simulink subsystem "rss_ActElecAgElecSpdCmptHybr"  (R2023a)
settings: Solver=VariableStepAuto  StartTime=0.0  StopTime=inf  RelTol=1e-3
undefined symbols (not defined in the file): bit, Cdbl_facPLLCtlKiMaxVal, Cdbl_facPLLCtlKpMaxVal, Cdbl_facVltgIntegFltCoeffMaxVal, Cdbl_indPhIndcMaxVal, Cdbl_indPhIndcPeakVal, Cdbl_iPhCurrMaxVal, Cdbl_iPhCurrPeakVal, Cdbl_nElecAgSpdMaxVal, Cdbl_nElecAgSpdPeakVal, Cdbl_psiPermMagFlxMaxVal, Cdbl_psiPermMagFlxPeakVal, Cdbl_resPhRstnMaxVal, Cdbl_resPhRstnPeakVal, Cdbl_tiMedTaskSmpTi, Cdbl_uPhVltgMaxVal, Cdbl_uSplyVltgPeakVal, dt_Standardize_s16p15b0, dt_Standardize_u16p15b0, ENM_MOTO_STATUS, Gs16_facPLLCtlKp_MAP_nActElecSpd_Y, Gs16_tiSenlElecAgDel_C, Gu16_facFlxObsFltCoeff_C, Gu16_facPLLCtlKi_MAP, Gu16_facPLLCtlKp_MAP, Gu16_indQaxIndc_C, Gu16_resPhRstn_C, Gu8_facPLLCtlKp_MAP_tPCBTempSubs_X, Gu8_numPPNum_C, lb_parOper6MaxVal, lb_parOper7MaxVal
libraries: lib_conversion x25, lib_discrete_time_integrator x5, lib_iir_filter x4, lib_configurable_parameter x3, lib_trigonometric_function x2, lib_finite_difference_derivative x2, simulink x1, lib_discrete_time_PI_controller32bit x1, lib_cart_to_polar_coor_transformer x1, lib_park_transform x1
settings Model: DefaultTestHarness=rss_ActualAngleAndSpeedComputation_thu  Creator=CAV2OFO  LastModifiedBy=xiaoqiang.yuan
settings OptimizationCC: ReuseModelBlockBuffer=off

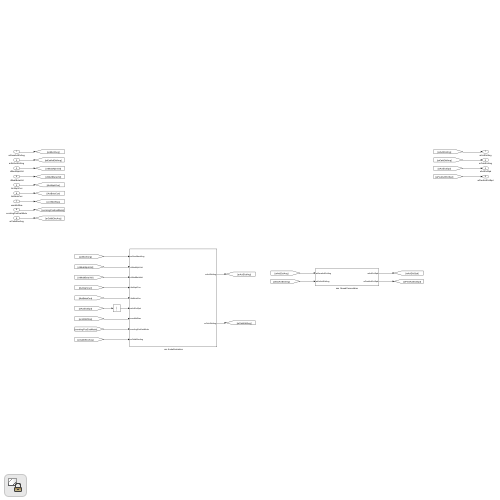
[thumbnail: Simulink's stored preview of the top-level diagram]
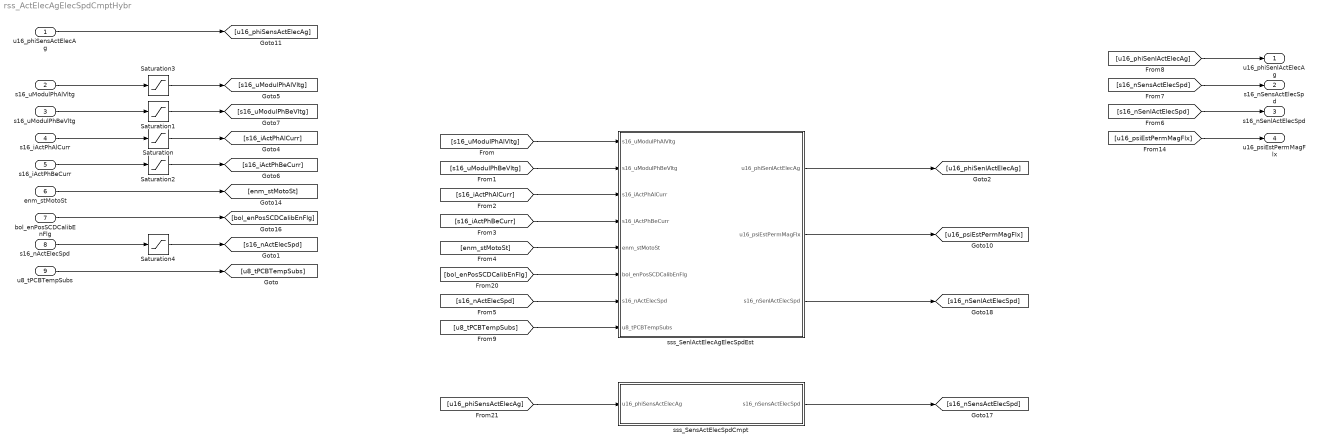
== system rss_ActElecAgElecSpdCmptHybr ==
  u16_phiSensActElecAg : Inport  OutDataTypeStr=dt_RadAng_u16r15b0
  s16_uModulPhAlVltg : Inport  Port=2  OutDataTypeStr=dt_Standardize_s16p15b0
  s16_uModulPhBeVltg : Inport  Port=3  OutDataTypeStr=dt_Standardize_s16p15b0
  s16_iActPhAlCurr : Inport  Port=4  OutDataTypeStr=dt_Standardize_s16p15b0
  s16_iActPhBeCurr : Inport  Port=5  OutDataTypeStr=dt_Standardize_s16p15b0
  enm_stMotoSt : Inport  Port=6  OutDataTypeStr=Enum: ENM_MOTO_STATUS
  bol_enPosSCDCalibEnFlg : Inport  Port=7  OutDataTypeStr=boolean
  s16_nActElecSpd : Inport  Port=8
  u8_tPCBTempSubs : Inport  Port=9
  Saturation : Saturate  UpperLimit=Cdbl_iPhCurrMaxVal  LowerLimit=-Cdbl_iPhCurrMaxVal
  Saturation1 : Saturate  UpperLimit=Cdbl_uPhVltgMaxVal  LowerLimit=-Cdbl_uPhVltgMaxVal
  Saturation2 : Saturate  UpperLimit=Cdbl_iPhCurrMaxVal  LowerLimit=-Cdbl_iPhCurrMaxVal
  Saturation3 : Saturate  UpperLimit=Cdbl_uPhVltgMaxVal  LowerLimit=-Cdbl_uPhVltgMaxVal
  Saturation4 : Saturate  UpperLimit=Cdbl_nElecAgSpdMaxVal  LowerLimit=-Cdbl_nElecAgSpdMaxVal
  sss_SenlActElecAgElecSpdEst : Subsystem
  sss_SensActElecSpdCmpt : Subsystem
  u16_phiSenlActElecAg : Outport  OutDataTypeStr=dt_RadAng_u16r15b0
  s16_nSensActElecSpd : Outport  Port=2  OutDataTypeStr=dt_Standardize_s16p15b0
  s16_nSenlActElecSpd : Outport  Port=3  OutDataTypeStr=dt_Standardize_s16p15b0  PortDimensions=1  VectorParamsAs1DForOutWhenUnconnected=off
  u16_psiEstPermMagFlx : Outport  Port=4  OutDataTypeStr=dt_Standardize_u16p15b0  PortDimensions=1  VectorParamsAs1DForOutWhenUnconnected=off
  wires:
  [s16_uModulPhAlVltg] -> sss_SenlActElecAgElecSpdEst/1(s16_uModulPhAlVltg)
  [s16_iActPhBeCurr] -> sss_SenlActElecAgElecSpdEst/4(s16_iActPhBeCurr)
  s16_iActPhBeCurr/1 -> Saturation2/1
  s16_iActPhAlCurr/1 -> Saturation/1
  [s16_iActPhAlCurr] -> sss_SenlActElecAgElecSpdEst/3(s16_iActPhAlCurr)
  sss_SenlActElecAgElecSpdEst/2(u16_psiEstPermMagFlx) -> [u16_psiEstPermMagFlx]
  [u16_psiEstPermMagFlx] -> u16_psiEstPermMagFlx/1
  [s16_uModulPhBeVltg] -> sss_SenlActElecAgElecSpdEst/2(s16_uModulPhBeVltg)
  s16_uModulPhBeVltg/1 -> Saturation1/1
  [u16_phiSenlActElecAg] -> u16_phiSenlActElecAg/1
  s16_uModulPhAlVltg/1 -> Saturation3/1
  [s16_nSensActElecSpd] -> s16_nSensActElecSpd/1
  enm_stMotoSt/1 -> [enm_stMotoSt]
  [enm_stMotoSt] -> sss_SenlActElecAgElecSpdEst/5(enm_stMotoSt)
  sss_SenlActElecAgElecSpdEst/1(u16_phiSenlActElecAg) -> [u16_phiSenlActElecAg]
  [s16_nSenlActElecSpd] -> s16_nSenlActElecSpd/1
  u16_phiSensActElecAg/1 -> [u16_phiSensActElecAg]
  bol_enPosSCDCalibEnFlg/1 -> [bol_enPosSCDCalibEnFlg]
  [bol_enPosSCDCalibEnFlg] -> sss_SenlActElecAgElecSpdEst/6(bol_enPosSCDCalibEnFlg)
  Saturation3/1 -> [s16_uModulPhAlVltg]
  Saturation1/1 -> [s16_uModulPhBeVltg]
  Saturation/1 -> [s16_iActPhAlCurr]
  Saturation2/1 -> [s16_iActPhBeCurr]
  [u16_phiSensActElecAg] -> sss_SensActElecSpdCmpt/1(u16_phiSensActElecAg)
  sss_SensActElecSpdCmpt/1(s16_nSensActElecSpd) -> [s16_nSensActElecSpd]
  sss_SenlActElecAgElecSpdEst/3(s16_nSenlActElecSpd) -> [s16_nSenlActElecSpd]
  s16_nActElecSpd/1 -> Saturation4/1
  [s16_nActElecSpd] -> sss_SenlActElecAgElecSpdEst/7(s16_nActElecSpd)
  Saturation4/1 -> [s16_nActElecSpd]
  [u8_tPCBTempSubs] -> sss_SenlActElecAgElecSpdEst/8(u8_tPCBTempSubs)
  u8_tPCBTempSubs/1 -> [u8_tPCBTempSubs]

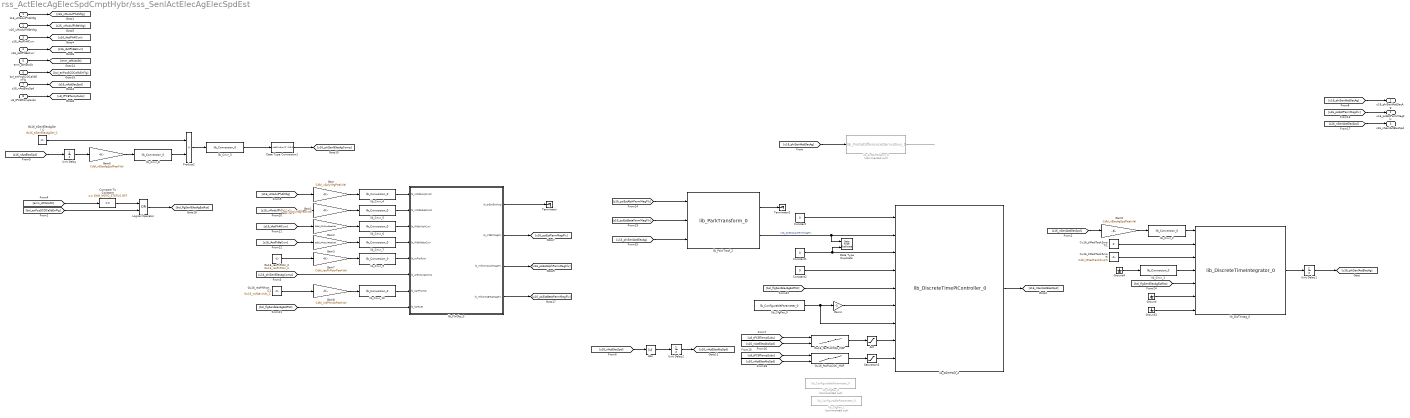
== system rss_ActElecAgElecSpdCmptHybr/sss_SenlActElecAgElecSpdEst ==
  s16_uModulPhAlVltg : Inport
  s16_uModulPhBeVltg : Inport  Port=2
  s16_iActPhAlCurr : Inport  Port=3
  s16_iActPhBeCurr : Inport  Port=4
  enm_stMotoSt : Inport  Port=5
  bol_enPosSCDCalibEnFlg : Inport  Port=6
  s16_nActElecSpd : Inport  Port=7
  u8_tPCBTempSubs : Inport  Port=8
  Abs : Abs  SaturateOnIntegerOverflow=off
  Ast : Saturate  UpperLimit=Cdbl_facPLLCtlKpMaxVal  LowerLimit=0
  Compare To Constant : simulink/Logic and Bit Operations/Compare To Constant  relop===  const=ENM_MOTO_STATUS.OFF  OutDataTypeStr=boolean
  Constant : Constant  Value=0  OutDataTypeStr=dt_Standardize_s16p15b0
  Constant1 : Constant  Value=0  OutDataTypeStr=Inherit: Inherit via back propagation
  Constant2 : Constant  Value=0  OutDataTypeStr=dt_Standardize_s16p15b0
  Cu16_tiMedTaskSmpTi : Constant  Value=Cdbl_tiMedTaskSmpTi
  Cu16_tiMedTaskSmpTi1 : Constant  Value=0  OutDataTypeStr=dt_RadAng_u16r15b0
  Data Type Duplicate : DataTypeDuplicate
  Data Type Conversion1 : DataTypeConversion  OutDataTypeStr=fixdt(0,16,pi*2^-15,0)  SaturateOnIntegerOverflow=off  RndMeth=Floor
  Gain : Gain  Gain=Cdbl_uSplyVltgPeakVal  OutDataTypeStr=Inherit: Inherit via back propagation
  Gain1 : Gain  Gain=Cdbl_uSplyVltgPeakVal  OutDataTypeStr=Inherit: Inherit via back propagation
  Gain2 : Gain  Gain=Cdbl_iPhCurrPeakVal  OutDataTypeStr=Inherit: Inherit via back propagation
  Gain3 : Gain  Gain=Cdbl_iPhCurrPeakVal  OutDataTypeStr=Inherit: Inherit via back propagation
  Gain4 : Gain  Gain=-1  OutDataTypeStr=Inherit: Same as input
  Gain5 : Gain  Gain=Cdbl_nElecAgSpdPeakVal  OutDataTypeStr=Inherit: Inherit via back propagation
  Gain6 : Gain  Gain=Cdbl_nElecAgSpdPeakVal  OutDataTypeStr=Inherit: Inherit via back propagation
  Gain7 : Gain  Gain=Cdbl_resPhRstnPeakVal  OutDataTypeStr=Inherit: Inherit via back propagation
  Gain8 : Gain  Gain=Cdbl_indPhIndcPeakVal  OutDataTypeStr=Inherit: Inherit via back propagation
  Ground : Ground
  Ground1 : Ground
  Ground4 : Ground
  Gs16_tiSenlElecAgDel_C : Constant  Value=Gs16_tiSenlElecAgDel_C
  Gu16_facPLLCtlKi_MAP : Lookup_n-D  BreakpointsForDimension1=Gu8_facPLLCtlKp_MAP_tPCBTempSubs_X  BreakpointsForDimension2=Gs16_facPLLCtlKp_MAP_nActElecSpd_Y  Table=Gu16_facPLLCtlKi_MAP  ExtrapMethod=Clip  InternalRulePriority=Speed  OutDataTypeStr=Inherit: Inherit from 'Table data'  RndMeth=Simplest  InputSameDT=off
      settings: InputPortMap=u0,u1
  Gu16_facPLLCtlKp_MAP : Lookup_n-D  BreakpointsForDimension1=Gu8_facPLLCtlKp_MAP_tPCBTempSubs_X  BreakpointsForDimension2=Gs16_facPLLCtlKp_MAP_nActElecSpd_Y  Table=Gu16_facPLLCtlKp_MAP  ExtrapMethod=Clip  InternalRulePriority=Speed  OutDataTypeStr=Inherit: Inherit from 'Table data'  RndMeth=Simplest  InputSameDT=off
      settings: InputPortMap=u0,u1
  Gu16_resPhRstn_C : Constant  Value=Gu16_resPhRstn_C
  Gu16_resPhRstn_C1 : Constant  Value=Gu16_indQaxIndc_C
  Logical Operator : Logic  Operator=OR  AllPortsSameDT=off  OutDataTypeStr=boolean
  Product2 : Product  OutDataTypeStr=Inherit: Inherit via back propagation
  Saturation3 : Saturate  UpperLimit=Cdbl_facPLLCtlKiMaxVal  LowerLimit=0
  Terminator : Terminator
  Terminator2 : Terminator
  Unit Delay : UnitDelay  SampleTime=-1  HasFrameUpgradeWarning=on
  Unit Delay1 : UnitDelay  SampleTime=-1  HasFrameUpgradeWarning=on
  Unit Delay2 : UnitDelay  SampleTime=-1  HasFrameUpgradeWarning=on
  lib_CfgPar_0 : lib_configurable_parameter/lib_ConfigurableParameter_0  lb_parCnfgPar=Gs16_nPLLElecAgSpdUpLim_C  lb_parDataType=Inherit: Inherit from 'Constant value'  lb_parUpLim=Cdbl_nElecAgSpdMaxVal  lb_parLowLim=0
  lib_CfgPar_1 : lib_configurable_parameter/lib_ConfigurableParameter_0  Commented=on  lb_parCnfgPar=Gu16_facPLLCtlKp_C  lb_parDataType=Inherit: Inherit from 'Constant value'  lb_parUpLim=Cdbl_facPLLCtlKpMaxVal  lb_parLowLim=0
  lib_CfgPar_2 : lib_configurable_parameter/lib_ConfigurableParameter_0  Commented=on  lb_parCnfgPar=Gu16_facPLLCtlKi_C  lb_parDataType=Inherit: Inherit from 'Constant value'  lb_parUpLim=Cdbl_facPLLCtlKiMaxVal  lb_parLowLim=0
  lib_Cnvr_1 : lib_conversion/lib_Conversion_0  lb_parDataType=uint8  lb_parOutpMaxVal=[]  lb_parOutpMinVal=[]  lb_parSatFlag=off
  lib_Cnvr_10 : lib_conversion/lib_Conversion_0  lb_parDataType=fixdt(0,16)  lb_parOutpMaxVal=Cdbl_indPhIndcPeakVal  lb_parOutpMinVal=[]  RndMeth=Simplest  lb_parSatFlag=off
  lib_Cnvr_2 : lib_conversion/lib_Conversion_0  lb_parDataType=fixdt(1,16)  lb_parOutpMaxVal=Cdbl_nElecAgSpdPeakVal  lb_parOutpMinVal=[]  RndMeth=Simplest  lb_parSatFlag=off
  lib_Cnvr_3 : lib_conversion/lib_Conversion_0  lb_parDataType=fixdt(1,16,pi*2^-15,0)  lb_parOutpMaxVal=[]  lb_parOutpMinVal=[]  lb_parSatFlag=off
  lib_Cnvr_4 : lib_conversion/lib_Conversion_0  lb_parDataType=fixdt(1,16)  lb_parOutpMaxVal=Cdbl_uSplyVltgPeakVal  lb_parOutpMinVal=[]  RndMeth=Simplest  lb_parSatFlag=off
  lib_Cnvr_5 : lib_conversion/lib_Conversion_0  lb_parDataType=fixdt(1,16)  lb_parOutpMaxVal=Cdbl_uSplyVltgPeakVal  lb_parOutpMinVal=[]  RndMeth=Simplest  lb_parSatFlag=off
  lib_Cnvr_6 : lib_conversion/lib_Conversion_0  lb_parDataType=fixdt(1,16)  lb_parOutpMaxVal=Cdbl_iPhCurrPeakVal  lb_parOutpMinVal=[]  RndMeth=Simplest  lb_parSatFlag=off
  lib_Cnvr_7 : lib_conversion/lib_Conversion_0  lb_parDataType=fixdt(1,16)  lb_parOutpMaxVal=Cdbl_iPhCurrPeakVal  lb_parOutpMinVal=[]  RndMeth=Simplest  lb_parSatFlag=off
  lib_Cnvr_8 : lib_conversion/lib_Conversion_0  lb_parDataType=fixdt(1,16)  lb_parOutpMaxVal=Cdbl_nElecAgSpdPeakVal  lb_parOutpMinVal=[]  RndMeth=Simplest  lb_parSatFlag=off
  lib_Cnvr_9 : lib_conversion/lib_Conversion_0  lb_parDataType=fixdt(0,16)  lb_parOutpMaxVal=Cdbl_resPhRstnPeakVal  lb_parOutpMinVal=[]  RndMeth=Simplest  lb_parSatFlag=off
  lib_DisTiInteg_0 : lib_discrete_time_integrator/lib_DiscreteTimeIntegrator_0  lb_parMaxInpVal=Cdbl_nElecAgSpdMaxVal*Cdbl_nElecAgSpdPeakVal  lb_parMinInpVal=-Cdbl_nElecAgSpdMaxVal*Cdbl_nElecAgSpdPeakVal  lb_parMaxSampTime=double(Cdbl_tiMedTaskSmpTi)  lb_parMaxIntgGain=0  lb_parAccmDataTypeMode=Same of output  lb_parOutpDataType=dt_RadAng_u16r15b0  lb_parIntgScopMode=Angular signal  lb_parSatFlag=off
  lib_DisTiPICtl_2 : lib_discrete_time_PI_controller32bit/lib_DiscreteTimePIController_0  lb_parSampTime=Cdbl_tiMedTaskSmpTi  lb_parMaxSampTime=0.1  lb_parMaxPropGain=Cdbl_facPLLCtlKpMaxVal  lb_parMaxIntgGain=Cdbl_facPLLCtlKiMaxVal  lb_parRefInpMaxVal=Cdbl_psiPermMagFlxMaxVal  lb_parRefInpMinVal=-Cdbl_psiPermMagFlxMaxVal  lb_parMaxErrVal=2*Cdbl_psiPermMagFlxMaxVal  lb_parMinErrVal=-2*Cdbl_psiPermMagFlxMaxVal  lb_parMaxOutpVal=Cdbl_nElecAgSpdMaxVal  lb_parMinOutpVal=-Cdbl_nElecAgSpdMaxVal  lb_parAccmDataTypeMode=32-bit  lb_parOutpDataType=dt_Standardize_s16p15b0  lb_parSatMode=anti-windup with back-calculation
  lib_FlxObs_0 : Subsystem  mask{lb_parPhsRstnMaxVal=Cdbl_resPhRstnMaxVal*Cdbl_resPhRstnPeakVal, lb_parPhsIndcMaxVal=Cdbl_indPhIndcMaxVal*Cdbl_indPhIndcPeakVal, lb_parPhsCurrMaxVal=Cdbl_iPhCurrMaxVal*Cdbl_iPhCurrPeakVal, lb_parPhsVoltMaxVal=Cdbl_uPhVltgMaxVal*Cdbl_uSplyVltgPeakVal, lb_parVoltIntgMaxVal=Cdbl_psiPermMagFlxMaxVal*Cdbl_psiPermMagFlxPeakVal*10, lb_parEstMagFluxMaxVal=Cdbl_psiPermMagFlxMaxVal*Cdbl_psiPermMagFlxPeakVal, lb_parPolePairNum=Gu8_numPPNum_C, lb_parSampTime=Cdbl_tiMedTaskSmpTi, lb_parFiltCoef=Gu16_facFlxObsFltCoeff_C, lb_parFltrCoefMaxVal=Cdbl_facVltgIntegFltCoeffMaxVal, lb_fluxPeak=Cdbl_psiPermMagFlxPeakVal, lb_parFluxAmpDataType=dt_Standardize_u16p15b0, lb_parFluxDataType=dt_Standardize_s16p15b0, lb_parBitNumMode=16-bit}
      mask prompts: lb_parPhsRstnMaxVal "Maximum phase resistance [Ohm]:"; lb_parPhsIndcMaxVal "Maximum phase inductance [H]:"; lb_parPhsCurrMaxVal "Maximum phase current [A]:"; lb_parPhsVoltMaxVal "Maximum phase voltage [V]:"; lb_parVoltIntgMaxVal "Maximum value for voltage integrator [Wb]:"; lb_parEstMagFluxMaxVal "Maximum estimated magnet flux [Wb]:"; lb_parPolePairNum "Number of pole pairs:"; lb_parSampTime "Sampling time [s]:"; lb_parFiltCoef "High-pass filter coefficient:"; lb_parFltrCoefMaxVal "High-pass filter coefficient maximum value:"; lb_fluxPeak "Peak output physical value[Wb]:"; lb_parFluxAmpDataType "Permanent magnet flux amplitude data type:"; lb_parFluxDataType "Permanent magnet flux data type:"; lb_parBitNumMode "Bits number for internal calculations:"
      mask init:
      | switch lb_parBitNumMode
      |     case '16-bit'
      |         lb_parBitNum = 16;
      |     case '32-bit'
      |         lb_parBitNum = 32;
      |     otherwise
      |         lb_parBitNum = 16;
      | end
      | 
      | % Operation 1: R*I
      | lb_parOper1MaxVal = lb_parPhsRstnMaxVal*lb_parPhsCurrMaxVal;
      | 
      | % Operation 2: V-R*I
      | lb_parOper2MaxVal = lb_parPhsVoltMaxVal+lb_parPhsRstnMaxVal*lb_parPhsCurrMaxVal;
      | 
      | % Operation 3: L*I
      | lb_parOper3MaxVal = lb_parPhsIndcMaxVal*lb_parPhsCurrMaxVal;
      | 
      | % Operation 4: integral of V-R*I
      | temp.oper4MaxVal = lb_parOper3MaxVal+lb_parEstMagFluxMaxVal;
      | lb_parIntgTurnOnThrs = lb_parVoltIntgMaxVal/2;
      | temp.intgMaxVal = lb_parVoltIntgMaxVal;
      | temp.NumType = fi(temp.intgMaxVal,1,lb_parBitNum);
      | lb_parIntgSlopExp = temp.NumType.FractionLength;
      | 
      | % Operation 5: filtering of flux
      | temp.NumType = fi(lb_parEstMagFluxMaxVal,1,16);
      | lb_parFiltSlopExp = temp.NumType.FractionLength;
      | 
      | % Operation 6: psi*I
      | %lb_parOper6MaxVal = lb_parPhsCurrMaxVal*lb_parEstMagFluxMaxVal;
      | 
      | % Operation 7: 2*psi*I
      | %lb_parOper7MaxVal = 2*lb_parPhsCurrMaxVal*lb_parEstMagFluxMaxVal;
      | 
      | % Operation 8: 3/2*Np
      | %lb_parOper8MaxVal = 3/2*double(lb_parPolePairNum);
      settings: LibrarySourceBlock=lib_flux_observer/lib_FluxObserver_0
      mask TypeOptions lb_parBitNumMode: 16-bit | 32-bit
      mask DialogControl DescGroupVar Prompt: Current Coupling block
      mask DialogControl DescTextVar Prompt: This block estimates electric angle, Permenant magnet flux and electric torque
      mask DialogControl modlPar Prompt: Model Parameters
      mask DialogControl Container3_copy Prompt: Data type:
      mask DialogControl Container3 Prompt: Operating modes:
  lib_FntDiffFltDrvt_0 : lib_finite_difference_derivative/lib_FiniteDifferenceDerivative_0  Commented=on  lb_parSampTime=Cdbl_tiMedTaskSmpTi  lb_parMaxInpVar=Cdbl_phiMaxMedTaskElecAgVrnt  lb_parOutpPhyPek=Cdbl_nElecAgSpdPeakVal  lb_parAngInpMode=on  lb_parOutpDataType=dt_Standardize_s16p15b0
      link override vss_AngleModeSelection: VariantControlMode=label  LabelModeActiveChoice=lb_parAngInpModeLbl
  lib_ParkTrasf_2 : lib_park_transform/lib_ParkTransform_0  VariantControl=ClarkTransf_MIL_flo  lb_parSelRotFrmeAxis=d-axis
  u16_phiSenlActElecAg : Outport
  u16_psiEstPermMagFlx : Outport  Port=2
  s16_nSenlActElecSpd : Outport  Port=3
  wires:
  Saturation3/1 -> lib_DisTiPICtl_2/9
  Ast/1 -> lib_DisTiPICtl_2/8
  [s16_nActElecAbsSpd] -> Gu16_facPLLCtlKi_MAP/2
  [s16_nActElecAbsSpd] -> Gu16_facPLLCtlKp_MAP/2
  Unit Delay2/1 -> [s16_nActElecAbsSpd]
  Gu16_facPLLCtlKi_MAP/1 -> Saturation3/1
  Gu16_facPLLCtlKp_MAP/1 -> Ast/1
  [u8_tPCBTempSubs] -> Gu16_facPLLCtlKi_MAP/1
  u8_tPCBTempSubs/1 -> [u8_tPCBTempSubs]
  [u8_tPCBTempSubs] -> Gu16_facPLLCtlKp_MAP/1
  Abs/1 -> Unit Delay2/1
  [s16_nActElecSpd] -> Abs/1
  [u16_phiSenlActElecAg] -> lib_FntDiffFltDrvt_0/1
  lib_FntDiffFltDrvt_0/1 -> ?
  s16_nActElecSpd/1 -> [s16_nActElecSpd]
  lib_FlxObs_0/4(lb_mfCompBetaMagFlx) -> [s16_psiEstBetaPermMagFlx]
  lib_FlxObs_0/3(lb_mfCompAlphMagFlx) -> [s16_psiEstAlphPermMagFlx]
  lib_Cnvr_10/1 -> lib_FlxObs_0/7(lb_parPhsIndc)
  Gain8/1 -> lib_Cnvr_10/1
  Gu16_resPhRstn_C1/1 -> Gain8/1
  Gu16_resPhRstn_C/1 -> Gain7/1
  lib_Cnvr_9/1 -> lib_FlxObs_0/5(lb_rsPhsRstn)
  Gain7/1 -> lib_Cnvr_9/1
  Unit Delay/1 -> Gain6/1
  lib_Cnvr_8/1 -> Product2/2
  Gain6/1 -> lib_Cnvr_8/1
  lib_DisTiPICtl_2/1 -> [s16_nSenlActElecSpd]
  Unit Delay1/1 -> [u16_phiSenlActElecAg]
  lib_Cnvr_2/1 -> lib_DisTiInteg_0/1
  Gain5/1 -> lib_Cnvr_2/1
  [s16_nSenlActElecSpd] -> Gain5/1
  Gain4/1 -> lib_DisTiPICtl_2/6
  lib_CfgPar_0/1 -> Gain4/1, lib_DisTiPICtl_2/7
  Ground1/1 -> lib_DisTiInteg_0/7
  Ground/1 -> lib_DisTiInteg_0/6
  [bol_flgSenlElecAgEstRst] -> lib_DisTiInteg_0/5
  lib_Cnvr_1/1 -> lib_DisTiInteg_0/4
  Cu16_tiMedTaskSmpTi1/1 -> lib_DisTiInteg_0/2
  Cu16_tiMedTaskSmpTi/1 -> lib_DisTiInteg_0/3
  Ground4/1 -> lib_Cnvr_1/1
  lib_DisTiInteg_0/1 -> Unit Delay1/1
  [bol_flgSenlElecAgEstRst] -> lib_DisTiPICtl_2/5
  [bol_flgSenlElecAgEstRst] -> lib_FlxObs_0/8(lb_bolRset)
  Logical Operator/1 -> [bol_flgSenlElecAgEstRst]
  Constant2/1 -> lib_DisTiPICtl_2/4
  Constant1/1 -> lib_DisTiPICtl_2/3, Data Type Duplicate/2
  lib_ParkTrasf_2/2 -> lib_DisTiPICtl_2/2, Data Type Duplicate/1  "s16_psiEstQaxPermMagFlx"
  lib_ParkTrasf_2/1 -> Terminator2/1
  Constant/1 -> lib_DisTiPICtl_2/1
  [u16_phiSenlActElecAg] -> lib_ParkTrasf_2/3
  [s16_psiEstBetaPermMagFlx] -> lib_ParkTrasf_2/2
  [s16_psiEstAlphPermMagFlx] -> lib_ParkTrasf_2/1
  [s16_nActElecSpd] -> Unit Delay/1
  [s16_nSenlActElecSpd] -> s16_nSenlActElecSpd/1
  [bol_enPosSCDCalibEnFlg] -> Logical Operator/2
  Compare To Constant/1 -> Logical Operator/1
  [u16_phiSenlElecAgComp] -> lib_FlxObs_0/6(lb_arElctAngComp)
  [s16_iActPhBeCurr] -> Gain3/1
  lib_Cnvr_4/1 -> lib_FlxObs_0/1(lb_vtFdbkAlphVolt)
  [s16_uModulPhAlVltg] -> Gain/1
  Gain3/1 -> lib_Cnvr_7/1
  lib_FlxObs_0/1(lb_arEstElctAng) -> Terminator/1
  lib_FlxObs_0/2(lb_mfEstMagFlx) -> [u16_psiEstPermMagFlx]
  [s16_iActPhAlCurr] -> Gain2/1
  Gain1/1 -> lib_Cnvr_5/1
  lib_Cnvr_6/1 -> lib_FlxObs_0/3(lb_iFdbkAlphCurr)
  Gain2/1 -> lib_Cnvr_6/1
  Gain/1 -> lib_Cnvr_4/1
  lib_Cnvr_7/1 -> lib_FlxObs_0/4(lb_iFdbkBetaCurr)
  [enm_stMotoSt] -> Compare To Constant/1
  lib_Cnvr_5/1 -> lib_FlxObs_0/2(lb_vtFdbkBetaVolt)
  [s16_uModulPhBeVltg] -> Gain1/1
  bol_enPosSCDCalibEnFlg/1 -> [bol_enPosSCDCalibEnFlg]
  s16_uModulPhBeVltg/1 -> [s16_uModulPhBeVltg]
  s16_uModulPhAlVltg/1 -> [s16_uModulPhAlVltg]
  enm_stMotoSt/1 -> [enm_stMotoSt]
  lib_Cnvr_3/1 -> Data Type Conversion1/1
  Data Type Conversion1/1 -> [u16_phiSenlElecAgComp]
  Product2/1 -> lib_Cnvr_3/1
  Gs16_tiSenlElecAgDel_C/1 -> Product2/1
  [u16_psiEstPermMagFlx] -> u16_psiEstPermMagFlx/1
  [u16_phiSenlActElecAg] -> u16_phiSenlActElecAg/1
  s16_iActPhBeCurr/1 -> [s16_iActPhBeCurr]
  s16_iActPhAlCurr/1 -> [s16_iActPhAlCurr]

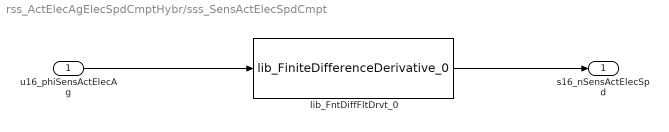
== system rss_ActElecAgElecSpdCmptHybr/sss_SensActElecSpdCmpt ==
  u16_phiSensActElecAg : Inport
  lib_FntDiffFltDrvt_0 : lib_finite_difference_derivative/lib_FiniteDifferenceDerivative_0  lb_parSampTime=Cdbl_tiMedTaskSmpTi  lb_parMaxInpVar=Cdbl_phiMaxMedTaskElecAgVrnt  lb_parOutpPhyPek=Cdbl_nElecAgSpdPeakVal  lb_parAngInpMode=on  lb_parOutpDataType=dt_Standardize_s16p15b0
      link override vss_AngleModeSelection: VariantControlMode=label  LabelModeActiveChoice=lb_parAngInpModeLbl
  s16_nSensActElecSpd : Outport
  wires:
  lib_FntDiffFltDrvt_0/1 -> s16_nSensActElecSpd/1
  u16_phiSensActElecAg/1 -> lib_FntDiffFltDrvt_0/1

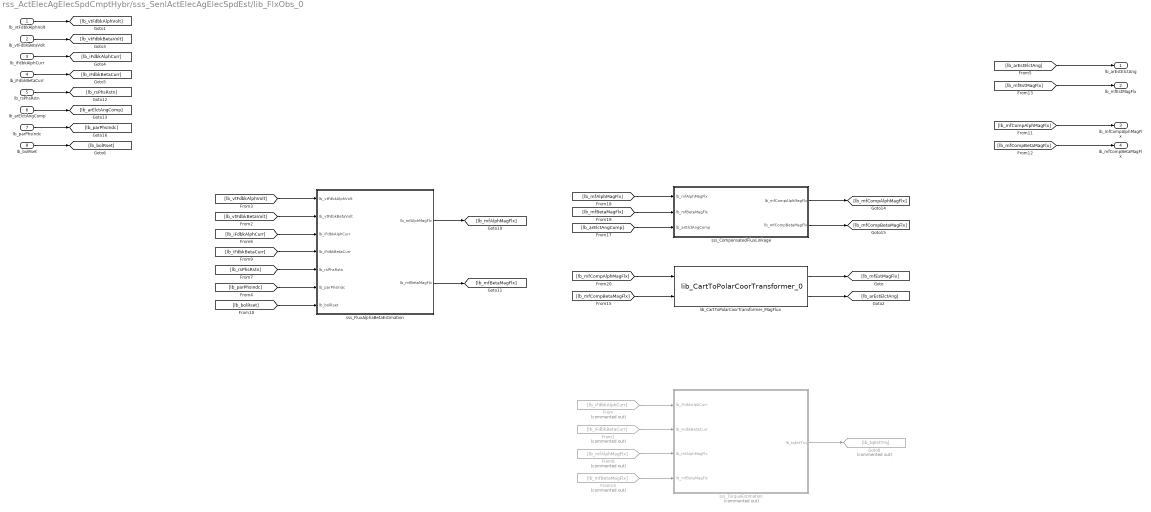
== system rss_ActElecAgElecSpdCmptHybr/sss_SenlActElecAgElecSpdEst/lib_FlxObs_0 ==
  lb_vtFdbkAlphVolt : Inport
  lb_vtFdbkBetaVolt : Inport  Port=2
  lb_iFdbkAlphCurr : Inport  Port=3
  lb_iFdbkBetaCurr : Inport  Port=4
  lb_rsPhsRstn : Inport  Port=5
  lb_arElctAngComp : Inport  Port=6  OutDataTypeStr=fixdt(0,16,pi*2^-15,0)
  lb_parPhsIndc : Inport  Port=7
  lb_bolRset : Inport  Port=8
  From : From  Commented=on  GotoTag=lb_iFdbkAlphCurr
  From1 : From  Commented=on  GotoTag=lb_iFdbkBetaCurr
  From14 : From  Commented=on  GotoTag=lb_mfBetaMagFlx
  From8 : From  Commented=on  GotoTag=lb_mfAlphMagFlx
  Goto8 : Goto  Commented=on  GotoTag=lb_tqEstTrq
  lib_CartToPolarCoorTransformer_MagFlux : lib_cart_to_polar_coor_transformer/lib_CartToPolarCoorTransformer_0  lb_parAsinLktSize=4095  lb_parAmpLktSize=512  lb_parOutpAmpDataType=lb_parFluxAmpDataType
      link override lib_MagnitudeCalculator_1/Compare To Constant/Compare: Operator===  OutDataTypeStr=boolean
      link override lib_MagnitudeCalculator_1/Compare To Constant1/Compare: Operator===  OutDataTypeStr=boolean
  sss_CompensatedFluxLinkage : Subsystem
  sss_FluxAlphaBetaEstimation : Subsystem
  sss_TorqueEstimation : Subsystem  Commented=on
  lb_arEstElctAng : Outport
  lb_mfEstMagFlx : Outport  Port=2
  lb_mfCompAlphMagFlx : Outport  Port=3
  lb_mfCompBetaMagFlx : Outport  Port=4
  wires:
  sss_CompensatedFluxLinkage/2(lb_mfCompBetaMagFlx) -> [lb_mfCompBetaMagFlx]
  sss_CompensatedFluxLinkage/1(lb_mfCompAlphMagFlx) -> [lb_mfCompAlphMagFlx]
  [lb_parPhsIndc] -> sss_FluxAlphaBetaEstimation/6(lb_parPhsIndc)
  lb_parPhsIndc/1 -> [lb_parPhsIndc]
  [lb_mfCompBetaMagFlx] -> lb_mfCompBetaMagFlx/1
  [lb_mfCompAlphMagFlx] -> lb_mfCompAlphMagFlx/1
  [lb_bolRset] -> sss_FluxAlphaBetaEstimation/7(lb_bolRset)
  lb_bolRset/1 -> [lb_bolRset]
  [lb_mfBetaMagFlx] -> sss_CompensatedFluxLinkage/2(lb_mfBetaMagFlx)
  [lb_mfAlphMagFlx] -> sss_CompensatedFluxLinkage/1(lb_mfAlphMagFlx)
  [lb_arElctAngComp] -> sss_CompensatedFluxLinkage/3(lb_arElctAngComp)
  lb_arElctAngComp/1 -> [lb_arElctAngComp]
  [lb_rsPhsRstn] -> sss_FluxAlphaBetaEstimation/5(lb_rsPhsRstn)
  lb_rsPhsRstn/1 -> [lb_rsPhsRstn]
  [lb_mfCompAlphMagFlx] -> lib_CartToPolarCoorTransformer_MagFlux/1
  [lb_mfCompBetaMagFlx] -> lib_CartToPolarCoorTransformer_MagFlux/2
  lib_CartToPolarCoorTransformer_MagFlux/2 -> [lb_arEstElctAng]
  From1/1 -> sss_TorqueEstimation/2(lb_iFdbkBetaCurr)
  From/1 -> sss_TorqueEstimation/1(lb_iFdbkAlphCurr)
  From14/1 -> sss_TorqueEstimation/4(lb_mfBetaMagFlx)
  From8/1 -> sss_TorqueEstimation/3(lb_mfAlphMagFlx)
  sss_FluxAlphaBetaEstimation/2(lb_mfBetaMagFlx) -> [lb_mfBetaMagFlx]
  sss_FluxAlphaBetaEstimation/1(lb_mfAlphMagFlx) -> [lb_mfAlphMagFlx]
  [lb_iFdbkBetaCurr] -> sss_FluxAlphaBetaEstimation/4(lb_iFdbkBetaCurr)
  [lb_vtFdbkBetaVolt] -> sss_FluxAlphaBetaEstimation/2(lb_vtFdbkBetaVolt)
  [lb_vtFdbkAlphVolt] -> sss_FluxAlphaBetaEstimation/1(lb_vtFdbkAlphVolt)
  lib_CartToPolarCoorTransformer_MagFlux/1 -> [lb_mfEstMagFlx]
  [lb_arEstElctAng] -> lb_arEstElctAng/1
  [lb_iFdbkAlphCurr] -> sss_FluxAlphaBetaEstimation/3(lb_iFdbkAlphCurr)
  lb_iFdbkAlphCurr/1 -> [lb_iFdbkAlphCurr]
  lb_vtFdbkBetaVolt/1 -> [lb_vtFdbkBetaVolt]
  sss_TorqueEstimation/1(lb_tqEstTrq) -> Goto8/1
  [lb_mfEstMagFlx] -> lb_mfEstMagFlx/1
  lb_iFdbkBetaCurr/1 -> [lb_iFdbkBetaCurr]
  lb_vtFdbkAlphVolt/1 -> [lb_vtFdbkAlphVolt]

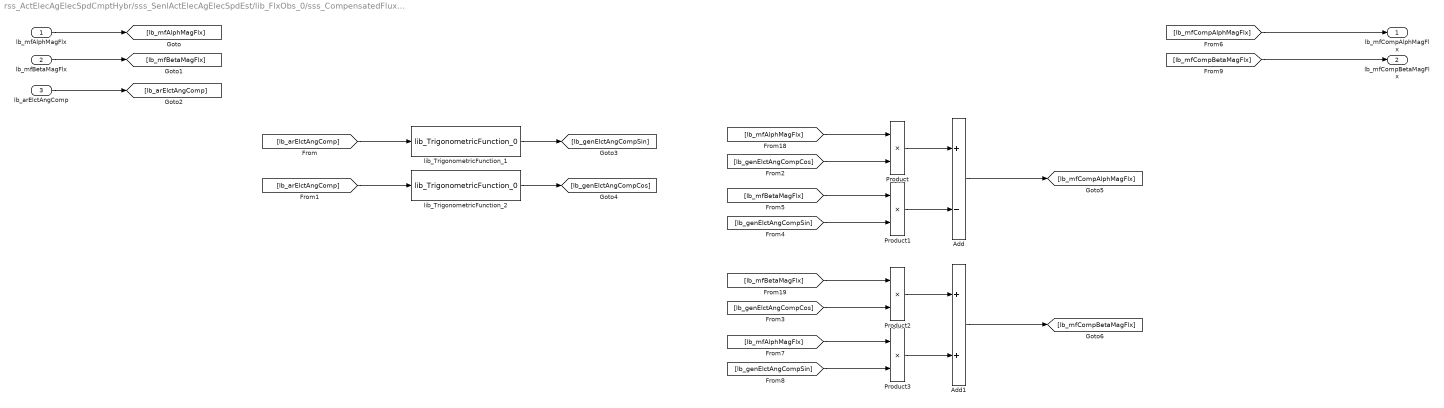
== system rss_ActElecAgElecSpdCmptHybr/sss_SenlActElecAgElecSpdEst/lib_FlxObs_0/sss_CompensatedFluxLinkage ==
  lb_mfAlphMagFlx : Inport
  lb_mfBetaMagFlx : Inport  Port=2
  lb_arElctAngComp : Inport  Port=3
  Add : Sum  Inputs=+-  OutDataTypeStr=Inherit: Same as first input
  Add1 : Sum  OutDataTypeStr=Inherit: Same as first input
  Product{,1..3} (4 alike) : Product  OutDataTypeStr=Inherit: Same as first input
  lib_TrigonometricFunction_1 : lib_trigonometric_function/lib_TrigonometricFunction_0  lb_parSelSigType=Sine  lb_parLktSizeStr=1024  lb_parOutpDataType=fixdt(1,16,2^-14,0)
  lib_TrigonometricFunction_2 : lib_trigonometric_function/lib_TrigonometricFunction_0  lb_parSelSigType=Cosine  lb_parLktSizeStr=1024  lb_parOutpDataType=fixdt(1,16,2^-14,0)
  lb_mfCompAlphMagFlx : Outport
  lb_mfCompBetaMagFlx : Outport  Port=2
  wires:
  [lb_mfCompBetaMagFlx] -> lb_mfCompBetaMagFlx/1
  [lb_mfCompAlphMagFlx] -> lb_mfCompAlphMagFlx/1
  Product2/1 -> Add1/1
  [lb_mfBetaMagFlx] -> Product2/1
  Product3/1 -> Add1/2
  Add1/1 -> [lb_mfCompBetaMagFlx]
  [lb_genElctAngCompSin] -> Product3/2
  [lb_genElctAngCompCos] -> Product2/2
  [lb_mfAlphMagFlx] -> Product3/1
  Add/1 -> [lb_mfCompAlphMagFlx]
  Product/1 -> Add/1
  Product1/1 -> Add/2
  [lb_mfBetaMagFlx] -> Product1/1
  [lb_genElctAngCompSin] -> Product1/2
  [lb_genElctAngCompCos] -> Product/2
  [lb_mfAlphMagFlx] -> Product/1
  lib_TrigonometricFunction_2/1 -> [lb_genElctAngCompCos]
  lib_TrigonometricFunction_1/1 -> [lb_genElctAngCompSin]
  [lb_arElctAngComp] -> lib_TrigonometricFunction_2/1
  [lb_arElctAngComp] -> lib_TrigonometricFunction_1/1
  lb_arElctAngComp/1 -> [lb_arElctAngComp]
  lb_mfBetaMagFlx/1 -> [lb_mfBetaMagFlx]
  lb_mfAlphMagFlx/1 -> [lb_mfAlphMagFlx]

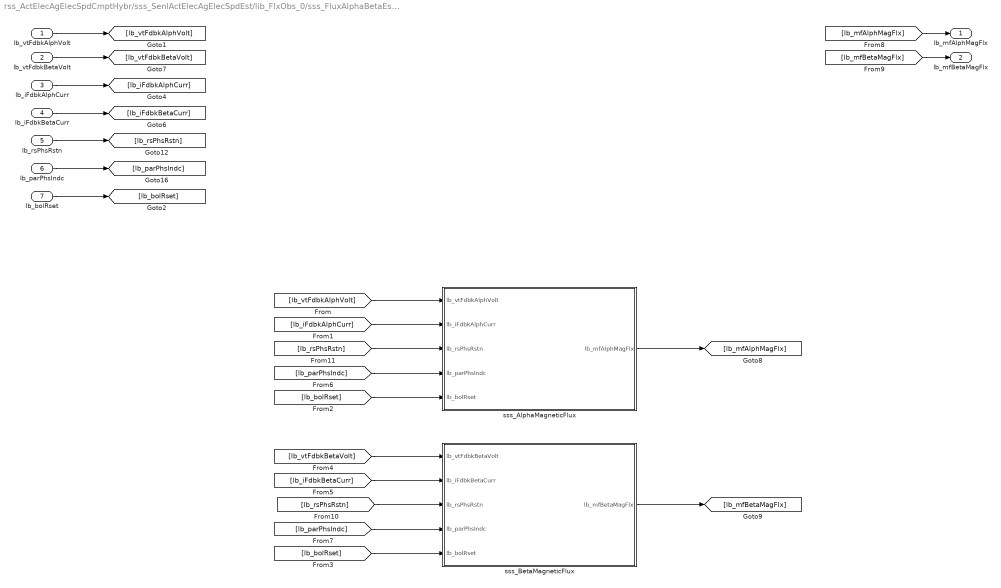
== system rss_ActElecAgElecSpdCmptHybr/sss_SenlActElecAgElecSpdEst/lib_FlxObs_0/sss_FluxAlphaBetaEstimation ==
  lb_vtFdbkAlphVolt : Inport
  lb_vtFdbkBetaVolt : Inport  Port=2
  lb_iFdbkAlphCurr : Inport  Port=3
  lb_iFdbkBetaCurr : Inport  Port=4
  lb_rsPhsRstn : Inport  Port=5
  lb_parPhsIndc : Inport  Port=6
  lb_bolRset : Inport  Port=7
  sss_AlphaMagneticFlux : Subsystem
  sss_BetaMagneticFlux : Subsystem
  lb_mfAlphMagFlx : Outport
  lb_mfBetaMagFlx : Outport  Port=2
  wires:
  [lb_parPhsIndc] -> sss_BetaMagneticFlux/4(lb_parPhsIndc)
  [lb_parPhsIndc] -> sss_AlphaMagneticFlux/4(lb_parPhsIndc)
  lb_parPhsIndc/1 -> [lb_parPhsIndc]
  [lb_bolRset] -> sss_BetaMagneticFlux/5(lb_bolRset)
  [lb_bolRset] -> sss_AlphaMagneticFlux/5(lb_bolRset)
  lb_bolRset/1 -> [lb_bolRset]
  sss_BetaMagneticFlux/1(lb_mfBetaMagFlx) -> [lb_mfBetaMagFlx]
  [lb_rsPhsRstn] -> sss_AlphaMagneticFlux/3(lb_rsPhsRstn)
  [lb_rsPhsRstn] -> sss_BetaMagneticFlux/3(lb_rsPhsRstn)
  lb_rsPhsRstn/1 -> [lb_rsPhsRstn]
  [lb_mfBetaMagFlx] -> lb_mfBetaMagFlx/1
  [lb_mfAlphMagFlx] -> lb_mfAlphMagFlx/1
  lb_vtFdbkBetaVolt/1 -> [lb_vtFdbkBetaVolt]
  lb_iFdbkBetaCurr/1 -> [lb_iFdbkBetaCurr]
  [lb_vtFdbkBetaVolt] -> sss_BetaMagneticFlux/1(lb_vtFdbkBetaVolt)
  [lb_iFdbkBetaCurr] -> sss_BetaMagneticFlux/2(lb_iFdbkBetaCurr)
  sss_AlphaMagneticFlux/1(lb_mfAlphMagFlx) -> [lb_mfAlphMagFlx]
  [lb_iFdbkAlphCurr] -> sss_AlphaMagneticFlux/2(lb_iFdbkAlphCurr)
  [lb_vtFdbkAlphVolt] -> sss_AlphaMagneticFlux/1(lb_vtFdbkAlphVolt)
  lb_vtFdbkAlphVolt/1 -> [lb_vtFdbkAlphVolt]
  lb_iFdbkAlphCurr/1 -> [lb_iFdbkAlphCurr]

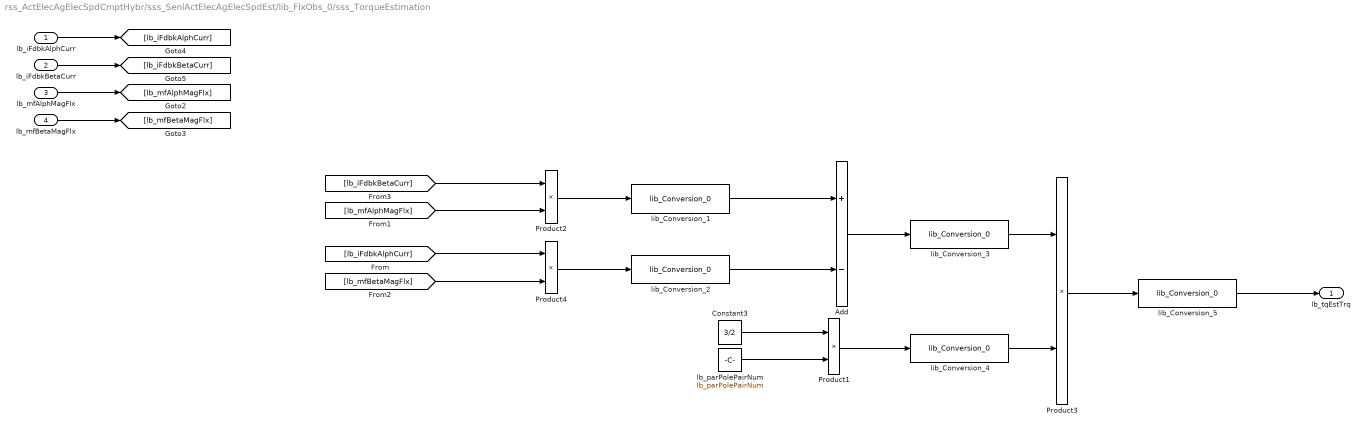
== system rss_ActElecAgElecSpdCmptHybr/sss_SenlActElecAgElecSpdEst/lib_FlxObs_0/sss_TorqueEstimation ==
  lb_iFdbkAlphCurr : Inport
  lb_iFdbkBetaCurr : Inport  Port=2
  lb_mfAlphMagFlx : Inport  Port=3
  lb_mfBetaMagFlx : Inport  Port=4
  Add : Sum  Inputs=+-  OutDataTypeStr=Inherit: Inherit via back propagation
  Constant3 : Constant  Value=3/2  OutDataTypeStr=fixdt(0,16,2^-15,0)
  Product{1..4} (4 alike) : Product  OutDataTypeStr=Inherit: Inherit via back propagation
  lb_parPolePairNum : Constant  Value=lb_parPolePairNum
  lib_Conversion_1 : lib_conversion/lib_Conversion_0  lb_parDataType=fixdt(1,16)  lb_parOutpMaxVal=lb_parOper6MaxVal  lb_parOutpMinVal=-lb_parOper6MaxVal  lb_parSatFlag=off
  lib_Conversion_2 : lib_conversion/lib_Conversion_0  lb_parDataType=fixdt(1,16)  lb_parOutpMaxVal=lb_parOper6MaxVal  lb_parOutpMinVal=-lb_parOper6MaxVal  lb_parSatFlag=off
  lib_Conversion_3 : lib_conversion/lib_Conversion_0  lb_parDataType=fixdt(1,16)  lb_parOutpMaxVal=lb_parOper7MaxVal  lb_parOutpMinVal=-lb_parOper7MaxVal  lb_parSatFlag=off
  lib_Conversion_4 : lib_conversion/lib_Conversion_0  lb_parDataType=fixdt(0,16)  lb_parOutpMaxVal=lb_parOper8MaxVal  lb_parOutpMinVal=[]  lb_parSatFlag=off
  lib_Conversion_5 : lib_conversion/lib_Conversion_0  lb_parDataType=lb_parMotTrqDataType  lb_parOutpMaxVal=[]  lb_parOutpMinVal=[]  lb_parSatFlag=off
  lb_tqEstTrq : Outport
  wires:
  lib_Conversion_2/1 -> Add/2
  Product4/1 -> lib_Conversion_2/1
  lib_Conversion_3/1 -> Product3/1
  lib_Conversion_4/1 -> Product3/2
  Product2/1 -> lib_Conversion_1/1
  lib_Conversion_1/1 -> Add/1
  Product1/1 -> lib_Conversion_4/1
  [lb_iFdbkBetaCurr] -> Product2/1
  [lb_mfAlphMagFlx] -> Product2/2
  [lb_iFdbkAlphCurr] -> Product4/1
  lb_iFdbkBetaCurr/1 -> [lb_iFdbkBetaCurr]
  lb_iFdbkAlphCurr/1 -> [lb_iFdbkAlphCurr]
  lb_parPolePairNum/1 -> Product1/2
  Constant3/1 -> Product1/1
  Add/1 -> lib_Conversion_3/1
  [lb_mfBetaMagFlx] -> Product4/2
  lib_Conversion_5/1 -> lb_tqEstTrq/1
  lb_mfBetaMagFlx/1 -> [lb_mfBetaMagFlx]
  lb_mfAlphMagFlx/1 -> [lb_mfAlphMagFlx]
  Product3/1 -> lib_Conversion_5/1

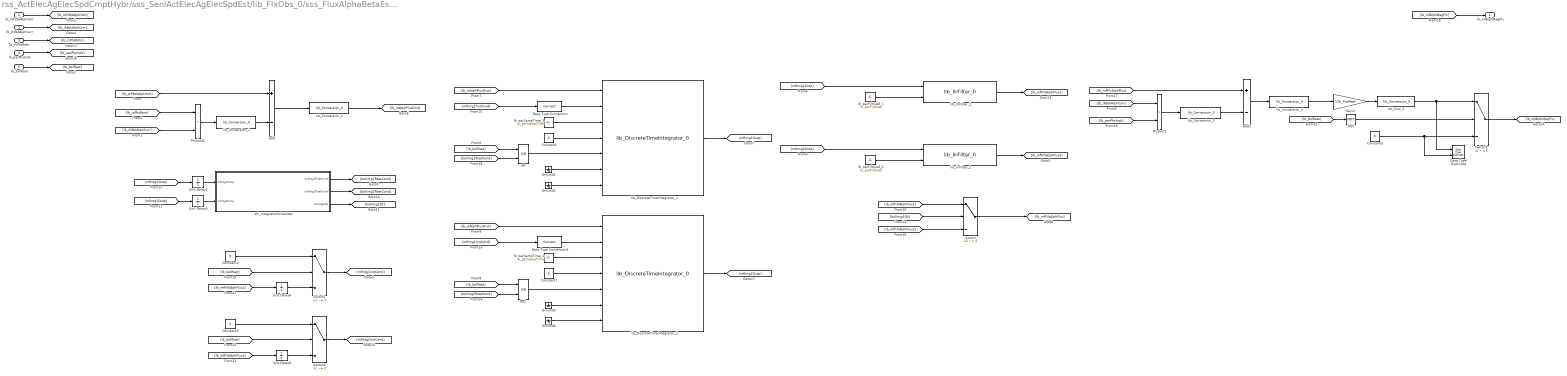
== system rss_ActElecAgElecSpdCmptHybr/sss_SenlActElecAgElecSpdEst/lib_FlxObs_0/sss_FluxAlphaBetaEstimation/sss_AlphaMagneticFlux ==
  lb_vtFdbkAlphVolt : Inport
  lb_iFdbkAlphCurr : Inport  Port=2
  lb_rsPhsRstn : Inport  Port=3
  lb_parPhsIndc : Inport  Port=4
  lb_bolRset : Inport  Port=5
  Add : Sum  Inputs=+-  OutDataTypeStr=Inherit: Inherit via back propagation
  Add1 : Sum  Inputs=+-  OutDataTypeStr=Inherit: Inherit via back propagation
  Constant : Constant  Value=0  OutDataTypeStr=uint8
  Constant1 : Constant  Value=0  OutDataTypeStr=uint8
  Constant2 : Constant  Value=0  OutDataTypeStr=fixdt(1,16,2^-lb_parFiltSlopExp,0)
  Constant3 : Constant  Value=0  OutDataTypeStr=fixdt(1,16,2^-lb_parFiltSlopExp,0)
  Constant5 : Constant  Value=0  OutDataTypeStr=Inherit: Inherit via back propagation
  Data Type Duplicate : DataTypeDuplicate
  Data Type Conversion : DataTypeConversion  SaturateOnIntegerOverflow=off  RndMeth=Floor
  Data Type Conversion1 : DataTypeConversion  SaturateOnIntegerOverflow=off  RndMeth=Floor
  Gain2 : Gain  Gain=1/lb_fluxPeak  OutDataTypeStr=Inherit: Inherit via back propagation
  Ground{1..4} (4 alike) : Ground
  NOT : Logic  Operator=NOT  AllPortsSameDT=off  OutDataTypeStr=boolean
  OR : Logic  Operator=OR  AllPortsSameDT=off  OutDataTypeStr=boolean
  OR1 : Logic  Operator=OR  AllPortsSameDT=off  OutDataTypeStr=boolean
  Product1 : Product  OutDataTypeStr=Inherit: Inherit via back propagation
  Product2 : Product  OutDataTypeStr=Inherit: Inherit via back propagation
  Switch{,1..3} (4 alike) : Switch  Criteria=u2 ~= 0  SaturateOnIntegerOverflow=off  InputSameDT=off
  Unit Delay{2..5} (4 alike) : UnitDelay  SampleTime=-1  HasFrameUpgradeWarning=on
  lb_parFiltCoef_1 : Constant  Value=lb_parFiltCoef
  lb_parFiltCoef_2 : Constant  Value=lb_parFiltCoef
  lb_parSampTime_1 : Constant  Value=lb_parSampTime
  lb_parSampTime_2 : Constant  Value=lb_parSampTime
  lib_Cnvr_1 : lib_conversion/lib_Conversion_0  lb_parDataType=lb_parFluxDataType  lb_parOutpMaxVal=[]  lb_parOutpMinVal=[]  lb_parSatFlag=off
  lib_Conversion_1 : lib_conversion/lib_Conversion_0  lb_parDataType=fixdt(1,lb_parBitNum)  lb_parOutpMaxVal=lb_parOper1MaxVal  lb_parOutpMinVal=-lb_parOper1MaxVal  lb_parSatFlag=off
  lib_Conversion_2 : lib_conversion/lib_Conversion_0  lb_parDataType=fixdt(1,lb_parBitNum)  lb_parOutpMaxVal=lb_parOper2MaxVal  lb_parOutpMinVal=-lb_parOper2MaxVal  lb_parSatFlag=off
  lib_Conversion_3 : lib_conversion/lib_Conversion_0  lb_parDataType=fixdt(1,lb_parBitNum)  lb_parOutpMaxVal=lb_parOper3MaxVal  lb_parOutpMinVal=-lb_parOper3MaxVal  lb_parSatFlag=off
  lib_Conversion_4 : lib_conversion/lib_Conversion_0  lb_parDataType=fixdt(1,16)  lb_parOutpMaxVal=lb_parEstMagFluxMaxVal  lb_parOutpMinVal=-lb_parEstMagFluxMaxVal  lb_parSatFlag=off
  lib_DiscreteTimeIntegrator_1 : lib_discrete_time_integrator/lib_DiscreteTimeIntegrator_0  lb_parMaxInpVal=lb_parOper2MaxVal  lb_parMinInpVal=-lb_parOper2MaxVal  lb_parMaxSampTime=double(lb_parSampTime)  lb_parMaxIntgGain=0  lb_parAccmDataTypeMode=Same of output  lb_parOutpDataType=fixdt(1,lb_parBitNum,2^-lb_parIntgSlopExp,0)  lb_parIntgScopMode=Generic signal  lb_parSatFlag=off
  lib_DiscreteTimeIntegrator_2 : lib_discrete_time_integrator/lib_DiscreteTimeIntegrator_0  lb_parMaxInpVal=lb_parOper2MaxVal  lb_parMinInpVal=-lb_parOper2MaxVal  lb_parMaxSampTime=double(lb_parSampTime)  lb_parMaxIntgGain=0  lb_parAccmDataTypeMode=Same of output  lb_parOutpDataType=fixdt(1,lb_parBitNum,2^-lb_parIntgSlopExp,0)  lb_parIntgScopMode=Generic signal  lb_parSatFlag=off
  lib_IirFilter_1 : lib_iir_filter/lib_IirFilter_0  lb_parMaxInpVal=lb_parVoltIntgMaxVal  lb_parFltrCoefMaxVal=lb_parFltrCoefMaxVal  lb_parBitNumMode=16-bit  lb_parOutpDataType=fixdt(1,16,2^-lb_parFiltSlopExp,0)  lb_parFiltTypeMode=High-pass
      link override vss_FilterVariant: VariantControlMode=label  LabelModeActiveChoice=lb_parHighPassModeLbl
  lib_IirFilter_2 : lib_iir_filter/lib_IirFilter_0  lb_parMaxInpVal=lb_parVoltIntgMaxVal  lb_parFltrCoefMaxVal=lb_parFltrCoefMaxVal  lb_parBitNumMode=16-bit  lb_parOutpDataType=fixdt(1,16,2^-lb_parFiltSlopExp,0)  lb_parFiltTypeMode=High-pass
      link override vss_FilterVariant: VariantControlMode=label  LabelModeActiveChoice=lb_parHighPassModeLbl
  sfc_IntegratorScheduler : Stateflow chart  TreatAsAtomicUnit=on
  lb_mfAlphMagFlx : Outport
  wires:
  [bolIntg2RsetCond] -> OR1/2
  [lb_bolRset] -> OR1/1
  OR1/1 -> lib_DiscreteTimeIntegrator_2/5
  [bolIntg1RsetCond] -> OR/2
  [lb_bolRset] -> OR/1
  OR/1 -> lib_DiscreteTimeIntegrator_1/5
  [lb_vtAlphFluxDrvt] -> lib_DiscreteTimeIntegrator_2/1
  [mfIntg2InitCond] -> Data Type Conversion1/1
  lb_parSampTime_2/1 -> lib_DiscreteTimeIntegrator_2/3
  Data Type Conversion1/1 -> lib_DiscreteTimeIntegrator_2/2
  lib_DiscreteTimeIntegrator_2/1 -> [mfIntg2Outp]
  Ground3/1 -> lib_DiscreteTimeIntegrator_2/6
  Ground4/1 -> lib_DiscreteTimeIntegrator_2/7
  Constant1/1 -> lib_DiscreteTimeIntegrator_2/4
  Switch/1 -> [lb_mfFiltAlphFlux]
  [bolIntg1Ok] -> Switch/2
  [lb_mfFiltAlphFlux1] -> Switch/1
  [lb_mfFiltAlphFlux2] -> Switch/3
  lb_parFiltCoef_2/1 -> lib_IirFilter_2/2
  lib_IirFilter_2/1 -> [lb_mfFiltAlphFlux2]
  [mfIntg2Outp] -> lib_IirFilter_2/1
  [lb_mfFiltAlphFlux1] -> Unit Delay5/1
  Switch1/1 -> [mfIntg1InitCond]
  Constant3/1 -> Switch2/1
  [lb_bolRset] -> Switch2/2
  [lb_bolRset] -> Switch1/2
  Unit Delay5/1 -> Switch2/3
  [lb_mfFiltAlphFlux2] -> Unit Delay4/1
  Constant2/1 -> Switch1/1
  Unit Delay4/1 -> Switch1/3
  Switch2/1 -> [mfIntg2InitCond]
  [mfIntg1Outp] -> Unit Delay2/1
  sfc_IntegratorScheduler/2(bolIntg2RsetCond) -> [bolIntg2RsetCond]
  sfc_IntegratorScheduler/1(bolIntg1RsetCond) -> [bolIntg1RsetCond]
  [mfIntg2Outp] -> Unit Delay3/1
  Unit Delay3/1 -> sfc_IntegratorScheduler/2(mfIntg2Outp)
  sfc_IntegratorScheduler/3(bolIntg1Ok) -> [bolIntg1Ok]
  Unit Delay2/1 -> sfc_IntegratorScheduler/1(mfIntg1Outp)
  Switch3/1 -> [lb_mfAlphMagFlx]
  [lb_vtAlphFluxDrvt] -> lib_DiscreteTimeIntegrator_1/1
  lb_parPhsIndc/1 -> [lb_parPhsIndc]
  lib_Conversion_4/1 -> Gain2/1
  lib_Cnvr_1/1 -> Switch3/1, Data Type Duplicate/1
  Gain2/1 -> lib_Cnvr_1/1
  NOT/1 -> Switch3/2
  Constant5/1 -> Switch3/3, Data Type Duplicate/2
  [lb_bolRset] -> NOT/1
  lb_bolRset/1 -> [lb_bolRset]
  [lb_mfAlphMagFlx] -> lb_mfAlphMagFlx/1
  [mfIntg1InitCond] -> Data Type Conversion/1
  [lb_mfFiltAlphFlux] -> Add1/1
  [mfIntg1Outp] -> lib_IirFilter_1/1
  lib_DiscreteTimeIntegrator_1/1 -> [mfIntg1Outp]
  lib_Conversion_2/1 -> [lb_vtAlphFluxDrvt]
  lib_IirFilter_1/1 -> [lb_mfFiltAlphFlux1]
  lb_parFiltCoef_1/1 -> lib_IirFilter_1/2
  Data Type Conversion/1 -> lib_DiscreteTimeIntegrator_1/2
  lib_Conversion_3/1 -> Add1/2
  Ground2/1 -> lib_DiscreteTimeIntegrator_1/7
  Constant/1 -> lib_DiscreteTimeIntegrator_1/4
  Ground1/1 -> lib_DiscreteTimeIntegrator_1/6
  lb_parSampTime_1/1 -> lib_DiscreteTimeIntegrator_1/3
  lib_Conversion_1/1 -> Add/2
  lb_rsPhsRstn/1 -> [lb_rsPhsRstn]
  Product1/1 -> lib_Conversion_1/1
  Add/1 -> lib_Conversion_2/1
  [lb_vtFdbkAlphVolt] -> Add/1
  lb_vtFdbkAlphVolt/1 -> [lb_vtFdbkAlphVolt]
  lb_iFdbkAlphCurr/1 -> [lb_iFdbkAlphCurr]
  [lb_iFdbkAlphCurr] -> Product1/2
  [lb_parPhsIndc] -> Product2/2
  [lb_rsPhsRstn] -> Product1/1
  [lb_iFdbkAlphCurr] -> Product2/1
  Product2/1 -> lib_Conversion_3/1
  Add1/1 -> lib_Conversion_4/1

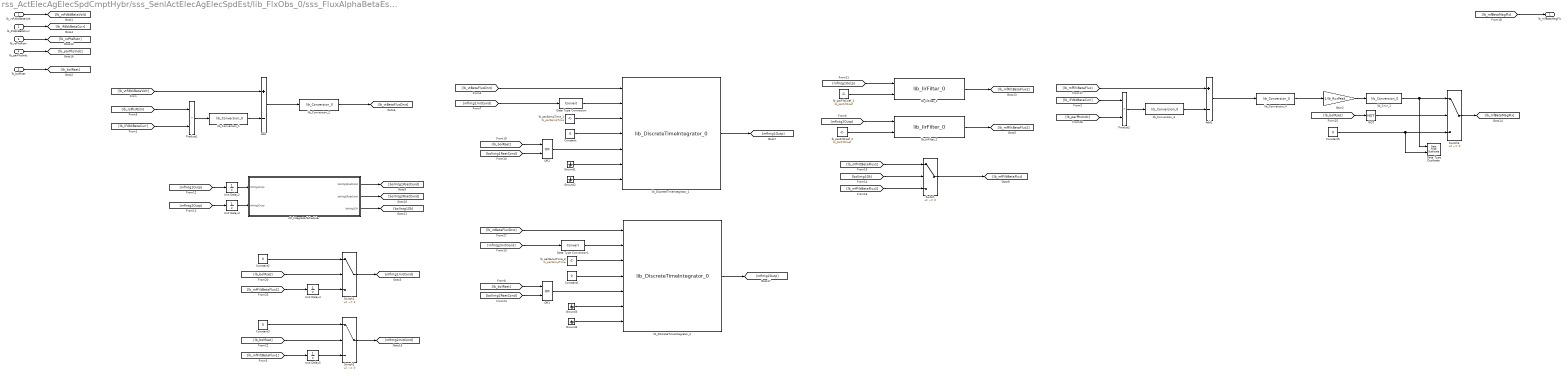
== system rss_ActElecAgElecSpdCmptHybr/sss_SenlActElecAgElecSpdEst/lib_FlxObs_0/sss_FluxAlphaBetaEstimation/sss_BetaMagneticFlux ==
  lb_vtFdbkBetaVolt : Inport
  lb_iFdbkBetaCurr : Inport  Port=2
  lb_rsPhsRstn : Inport  Port=3
  lb_parPhsIndc : Inport  Port=4
  lb_bolRset : Inport  Port=5
  Add : Sum  Inputs=+-  OutDataTypeStr=Inherit: Inherit via back propagation
  Add1 : Sum  Inputs=+-  OutDataTypeStr=Inherit: Inherit via back propagation
  Constant : Constant  Value=0  OutDataTypeStr=uint8
  Constant1 : Constant  Value=0  OutDataTypeStr=uint8
  Constant2 : Constant  Value=0  OutDataTypeStr=fixdt(1,16,2^-lb_parFiltSlopExp,0)
  Constant3 : Constant  Value=0  OutDataTypeStr=fixdt(1,16,2^-lb_parFiltSlopExp,0)
  Constant5 : Constant  Value=0  OutDataTypeStr=Inherit: Inherit via back propagation
  Data Type Duplicate : DataTypeDuplicate
  Data Type Conversion : DataTypeConversion  SaturateOnIntegerOverflow=off  RndMeth=Floor
  Data Type Conversion1 : DataTypeConversion  SaturateOnIntegerOverflow=off  RndMeth=Floor
  Gain2 : Gain  Gain=1/lb_fluxPeak  OutDataTypeStr=Inherit: Inherit via back propagation
  Ground{1..4} (4 alike) : Ground
  NOT : Logic  Operator=NOT  AllPortsSameDT=off  OutDataTypeStr=boolean
  OR1 : Logic  Operator=OR  AllPortsSameDT=off  OutDataTypeStr=boolean
  OR2 : Logic  Operator=OR  AllPortsSameDT=off  OutDataTypeStr=boolean
  Product1 : Product  OutDataTypeStr=Inherit: Inherit via back propagation
  Product2 : Product  OutDataTypeStr=Inherit: Inherit via back propagation
  Switch{,1..3} (4 alike) : Switch  Criteria=u2 ~= 0  SaturateOnIntegerOverflow=off  InputSameDT=off
  Unit Delay{2..5} (4 alike) : UnitDelay  SampleTime=-1  HasFrameUpgradeWarning=on
  lb_parFiltCoef_1 : Constant  Value=lb_parFiltCoef
  lb_parFiltCoef_2 : Constant  Value=lb_parFiltCoef
  lb_parSampTime_1 : Constant  Value=lb_parSampTime
  lb_parSampTime_2 : Constant  Value=lb_parSampTime
  lib_Cnvr_1 : lib_conversion/lib_Conversion_0  lb_parDataType=lb_parFluxDataType  lb_parOutpMaxVal=[]  lb_parOutpMinVal=[]  lb_parSatFlag=off
  lib_Conversion_1 : lib_conversion/lib_Conversion_0  lb_parDataType=fixdt(1,lb_parBitNum)  lb_parOutpMaxVal=lb_parOper1MaxVal  lb_parOutpMinVal=-lb_parOper1MaxVal  lb_parSatFlag=off
  lib_Conversion_2 : lib_conversion/lib_Conversion_0  lb_parDataType=fixdt(1,lb_parBitNum)  lb_parOutpMaxVal=lb_parOper2MaxVal  lb_parOutpMinVal=-lb_parOper2MaxVal  lb_parSatFlag=off
  lib_Conversion_3 : lib_conversion/lib_Conversion_0  lb_parDataType=fixdt(1,lb_parBitNum)  lb_parOutpMaxVal=lb_parOper3MaxVal  lb_parOutpMinVal=-lb_parOper3MaxVal  lb_parSatFlag=off
  lib_Conversion_4 : lib_conversion/lib_Conversion_0  lb_parDataType=fixdt(1,16)  lb_parOutpMaxVal=lb_parEstMagFluxMaxVal  lb_parOutpMinVal=-lb_parEstMagFluxMaxVal  lb_parSatFlag=off
  lib_DiscreteTimeIntegrator_1 : lib_discrete_time_integrator/lib_DiscreteTimeIntegrator_0  lb_parMaxInpVal=lb_parOper2MaxVal  lb_parMinInpVal=-lb_parOper2MaxVal  lb_parMaxSampTime=double(lb_parSampTime)  lb_parMaxIntgGain=0  lb_parAccmDataTypeMode=Same of output  lb_parOutpDataType=fixdt(1,lb_parBitNum,2^-lb_parIntgSlopExp,0)  lb_parIntgScopMode=Generic signal  lb_parSatFlag=off
  lib_DiscreteTimeIntegrator_2 : lib_discrete_time_integrator/lib_DiscreteTimeIntegrator_0  lb_parMaxInpVal=lb_parOper2MaxVal  lb_parMinInpVal=-lb_parOper2MaxVal  lb_parMaxSampTime=double(lb_parSampTime)  lb_parMaxIntgGain=0  lb_parAccmDataTypeMode=Same of output  lb_parOutpDataType=fixdt(1,lb_parBitNum,2^-lb_parIntgSlopExp,0)  lb_parIntgScopMode=Generic signal  lb_parSatFlag=off
  lib_IirFilter_1 : lib_iir_filter/lib_IirFilter_0  lb_parMaxInpVal=lb_parVoltIntgMaxVal  lb_parFltrCoefMaxVal=lb_parFltrCoefMaxVal  lb_parBitNumMode=16-bit  lb_parOutpDataType=fixdt(1,16,2^-lb_parFiltSlopExp,0)  lb_parFiltTypeMode=High-pass
      link override vss_FilterVariant: VariantControlMode=label  LabelModeActiveChoice=lb_parHighPassModeLbl
  lib_IirFilter_2 : lib_iir_filter/lib_IirFilter_0  lb_parMaxInpVal=lb_parVoltIntgMaxVal  lb_parFltrCoefMaxVal=lb_parFltrCoefMaxVal  lb_parBitNumMode=16-bit  lb_parOutpDataType=fixdt(1,16,2^-lb_parFiltSlopExp,0)  lb_parFiltTypeMode=High-pass
      link override vss_FilterVariant: VariantControlMode=label  LabelModeActiveChoice=lb_parHighPassModeLbl
  sfc_IntegratorScheduler : Stateflow chart  TreatAsAtomicUnit=on
  lb_mfBetaMagFlx : Outport
  wires:
  [bolIntg1RsetCond] -> OR2/2
  [lb_bolRset] -> OR2/1
  OR2/1 -> lib_DiscreteTimeIntegrator_1/5
  [lb_vtBetaFluxDrvt] -> lib_DiscreteTimeIntegrator_2/1
  Unit Delay2/1 -> sfc_IntegratorScheduler/1(mfIntg1Outp)
  [bolIntg2RsetCond] -> OR1/2
  OR1/1 -> lib_DiscreteTimeIntegrator_2/5
  Unit Delay4/1 -> Switch1/3
  [lb_bolRset] -> Switch1/2
  Switch2/1 -> [mfIntg2InitCond]
  sfc_IntegratorScheduler/1(bolIntg1RsetCond) -> [bolIntg1RsetCond]
  Constant2/1 -> Switch1/1
  sfc_IntegratorScheduler/3(bolIntg1Ok) -> [bolIntg1Ok]
  sfc_IntegratorScheduler/2(bolIntg2RsetCond) -> [bolIntg2RsetCond]
  [mfIntg2Outp] -> Unit Delay3/1
  [mfIntg2Outp] -> lib_IirFilter_2/1
  [lb_mfFiltBetaFlux2] -> Unit Delay4/1
  Constant1/1 -> lib_DiscreteTimeIntegrator_2/4
  Switch1/1 -> [mfIntg1InitCond]
  lb_parFiltCoef_2/1 -> lib_IirFilter_2/2
  Constant3/1 -> Switch2/1
  Unit Delay3/1 -> sfc_IntegratorScheduler/2(mfIntg2Outp)
  Ground4/1 -> lib_DiscreteTimeIntegrator_2/7
  [mfIntg1Outp] -> Unit Delay2/1
  Switch/1 -> [lb_mfFiltBetaFlux]
  Ground3/1 -> lib_DiscreteTimeIntegrator_2/6
  [bolIntg1Ok] -> Switch/2
  Unit Delay5/1 -> Switch2/3
  lib_IirFilter_2/1 -> [lb_mfFiltBetaFlux2]
  [mfIntg2InitCond] -> Data Type Conversion1/1
  [lb_mfFiltBetaFlux2] -> Switch/3
  lb_parSampTime_2/1 -> lib_DiscreteTimeIntegrator_2/3
  [lb_mfFiltBetaFlux1] -> Unit Delay5/1
  [lb_bolRset] -> Switch2/2
  lib_DiscreteTimeIntegrator_2/1 -> [mfIntg2Outp]
  Data Type Conversion1/1 -> lib_DiscreteTimeIntegrator_2/2
  [lb_mfFiltBetaFlux1] -> Switch/1
  [lb_bolRset] -> OR1/1
  Switch3/1 -> [lb_mfBetaMagFlx]
  lib_DiscreteTimeIntegrator_1/1 -> [mfIntg1Outp]
  lb_parPhsIndc/1 -> [lb_parPhsIndc]
  lib_Cnvr_1/1 -> Switch3/1, Data Type Duplicate/1
  lib_Conversion_4/1 -> Gain2/1
  Gain2/1 -> lib_Cnvr_1/1
  Constant5/1 -> Switch3/3, Data Type Duplicate/2
  NOT/1 -> Switch3/2
  [lb_bolRset] -> NOT/1
  [mfIntg1InitCond] -> Data Type Conversion/1
  lb_bolRset/1 -> [lb_bolRset]
  [lb_mfBetaMagFlx] -> lb_mfBetaMagFlx/1
  [lb_mfFiltBetaFlux] -> Add1/1
  [mfIntg1Outp] -> lib_IirFilter_1/1
  [lb_vtBetaFluxDrvt] -> lib_DiscreteTimeIntegrator_1/1
  lib_Conversion_2/1 -> [lb_vtBetaFluxDrvt]
  lib_IirFilter_1/1 -> [lb_mfFiltBetaFlux1]
  lb_parFiltCoef_1/1 -> lib_IirFilter_1/2
  Data Type Conversion/1 -> lib_DiscreteTimeIntegrator_1/2
  lib_Conversion_3/1 -> Add1/2
  Ground2/1 -> lib_DiscreteTimeIntegrator_1/7
  Constant/1 -> lib_DiscreteTimeIntegrator_1/4
  Ground1/1 -> lib_DiscreteTimeIntegrator_1/6
  lb_parSampTime_1/1 -> lib_DiscreteTimeIntegrator_1/3
  lib_Conversion_1/1 -> Add/2
  lb_rsPhsRstn/1 -> [lb_rsPhsRstn]
  Product1/1 -> lib_Conversion_1/1
  Add/1 -> lib_Conversion_2/1
  [lb_vtFdbkBetaVolt] -> Add/1
  lb_vtFdbkBetaVolt/1 -> [lb_vtFdbkBetaVolt]
  lb_iFdbkBetaCurr/1 -> [lb_iFdbkBetaCurr]
  [lb_iFdbkBetaCurr] -> Product1/2
  [lb_parPhsIndc] -> Product2/2
  [lb_rsPhsRstn] -> Product1/1
  [lb_iFdbkBetaCurr] -> Product2/1
  Product2/1 -> lib_Conversion_3/1
  Add1/1 -> lib_Conversion_4/1

== stateflow chart rss_ActElecAgElecSpdCmptHybr/sss_SenlActElecAgElecSpdEst/lib_FlxObs_0/sss_FluxAlphaBetaEstimation/sss_BetaMagneticFlux/sfc_IntegratorScheduler ==
  state INTG1ON_INTG2ON
    en:
    bolIntg1RsetCond = false;
    bolIntg2RsetCond = false;
  state INTG1OFF_INTG2ON
    en:
    bolIntg1RsetCond = true;
    bolIntg2RsetCond = false;
    bolIntg1Ok = false;
  state INTG1ON_INTG2OFF
    en:
    bolIntg1RsetCond = false;
    bolIntg2RsetCond = true;
    bolIntg1Ok = true;
  (default) -> INTG1ON_INTG2OFF
  INTG1OFF_INTG2ON -> INTG1ON_INTG2ON : [abs(mfIntg2Outp) >= abs(lb_parIntgTurnOnThrs)]
  INTG1ON_INTG2ON -> INTG1ON_INTG2OFF [order 2] : [after(300,tick) && ~bolIntg1Ok]
  INTG1ON_INTG2ON -> INTG1OFF_INTG2ON [order 1] : [after(300,tick) && bolIntg1Ok]
  INTG1ON_INTG2OFF -> INTG1ON_INTG2ON : [abs(mfIntg1Outp) >= abs(lb_parIntgTurnOnThrs)]
  data: mfIntg1Outp input; mfIntg2Outp input; bolIntg1RsetCond output boolean; bolIntg2RsetCond output boolean; lb_parIntgTurnOnThrs parameter fixdt(1,lb_parBitNum,2^-lb_parIntgSlopExp,0); bolIntg1Ok output boolean

== stateflow chart rss_ActElecAgElecSpdCmptHybr/sss_SenlActElecAgElecSpdEst/lib_FlxObs_0/sss_FluxAlphaBetaEstimation/sss_AlphaMagneticFlux/sfc_IntegratorScheduler ==
  state INTG1ON_INTG2ON
    en:
    bolIntg1RsetCond = false;
    bolIntg2RsetCond = false;
  state INTG1OFF_INTG2ON
    en:
    bolIntg1RsetCond = true;
    bolIntg2RsetCond = false;
    bolIntg1Ok = false;
  state INTG1ON_INTG2OFF
    en:
    bolIntg1RsetCond = false;
    bolIntg2RsetCond = true;
    bolIntg1Ok = true;
  (default) -> INTG1ON_INTG2OFF
  INTG1OFF_INTG2ON -> INTG1ON_INTG2ON : [abs(mfIntg2Outp) >= abs(lb_parIntgTurnOnThrs)]
  INTG1ON_INTG2ON -> INTG1ON_INTG2OFF [order 2] : [after(300,tick) && ~bolIntg1Ok]
  INTG1ON_INTG2ON -> INTG1OFF_INTG2ON [order 1] : [after(300,tick) && bolIntg1Ok]
  INTG1ON_INTG2OFF -> INTG1ON_INTG2ON : [abs(mfIntg1Outp) >= abs(lb_parIntgTurnOnThrs)]
  data: mfIntg1Outp input; mfIntg2Outp input; bolIntg1RsetCond output boolean; bolIntg2RsetCond output boolean; lb_parIntgTurnOnThrs parameter fixdt(1,lb_parBitNum,2^-lb_parIntgSlopExp,0); bolIntg1Ok output boolean
